simulink subsystem "PvtSubSys_VSM_LKA"  (R2020b)
settings: Solver=VariableStepAuto  StartTime=0.0  StopTime=10.0  RelTol=1e-3
values from neighbouring files (symbols this model uses):
  P_VSM_LKA_AbsEspInTime = 3.0    [LKA.sldd]
  P_VSM_LKA_absLongitudeAcceIn = 2.5    [LKA.sldd]
  P_VSM_LKA_absLongitudeAcceInTime = 3.0    [LKA.sldd]
  P_VSM_LKA_absLongitudeAcceOut = 3.0    [LKA.sldd]
  P_VSM_LKA_AccPedalPosnOut = 30.0    [LKA.sldd]
  P_VSM_LKA_AccPedalRateOutTime = 0.0    [LKA.sldd]
  P_VSM_LKA_AccRateIn = 30.0    [LKA.sldd]
  P_VSM_LKA_AccRateInTime = 1.5    [LKA.sldd]
  P_VSM_LKA_AccRateOut = 70.0    [LKA.sldd]
  P_VSM_LKA_BrakePressIn = 3.0    [LKA.sldd]
  P_VSM_LKA_BrakePressInTime = 1.5    [LKA.sldd]
  P_VSM_LKA_BrakePressOut = 5.0    [LKA.sldd]
  P_VSM_LKA_CurveFactor = 1.0    [LKA.sldd]
  P_VSM_LKA_DriverInputTrqValueIn = 2.0    [LKA.sldd]
  P_VSM_LKA_DriverInputTrqValueInTime = 3.0    [LKA.sldd]
  P_VSM_LKA_DriverInputTrqValueOut = 2.3    [LKA.sldd]
  P_VSM_LKA_EndSwitch = 1.0    [LKA.sldd]
  P_VSM_LKA_LaneChangeOffset = 0.11    [LKA.sldd]
  P_VSM_LKA_LaneCurveIn = 0.005    [LKA.sldd]
  P_VSM_LKA_LaneCurveOut = 0.006    [LKA.sldd]
  P_VSM_LKA_LateralAcceIn = 3.0    [LKA.sldd]
  P_VSM_LKA_LateralAcceInTime = 3.0    [LKA.sldd]
  P_VSM_LKA_LateralAcceOut = 3.5    [LKA.sldd]
  P_VSM_LKA_LongitudeAcceIn = 3.0    [LKA.sldd]
  P_VSM_LKA_LongitudeAcceOut = 3.5    [LKA.sldd]
  P_VSM_LKA_OverrideInTime = 1.5    [LKA.sldd]
  P_VSM_LKA_OverrideTime = 0.3    [LKA.sldd]
  P_VSM_LKA_OverrideValue = 1.2    [LKA.sldd]
  P_VSM_LKA_State_Absesp_enable = 1.0    [LKA.sldd]
  P_VSM_LKA_State_Accpedalrate_enable = 1.0    [LKA.sldd]
  P_VSM_LKA_State_Breakpressure_enable = 1.0    [LKA.sldd]
  P_VSM_LKA_State_DriverInputTrqValue_enable = 1.0    [LKA.sldd]
  P_VSM_LKA_State_Eps_enable = 1.0    [LKA.sldd]
  P_VSM_LKA_State_ESSSts_enable = 1.0    [LKA.sldd]
  P_VSM_LKA_State_Failsafe_enable = 1.0    [LKA.sldd]
  P_VSM_LKA_State_GEAR_enable = 1.0    [LKA.sldd]
  P_VSM_LKA_State_Handson_enable = 1.0    [LKA.sldd]
  P_VSM_LKA_State_Headingangle_enable = 1.0    [LKA.sldd]
  P_VSM_LKA_State_Lane_enable = 1.0    [LKA.sldd]
  P_VSM_LKA_State_LaneChange_enable = 1.0    [LKA.sldd]
  P_VSM_LKA_State_Lanecurve_enable = 1.0    [LKA.sldd]
  P_VSM_LKA_State_LateralAcce_enable = 1.0    [LKA.sldd]
  P_VSM_LKA_State_LongitudeAcc_enable = 1.0    [LKA.sldd]
  P_VSM_LKA_State_Overide_enable = 1.0    [LKA.sldd]
  P_VSM_LKA_State_Param_AngleOffset = 0.15    [LKA.sldd]
  P_VSM_LKA_State_Param_InterventionZoneIn = 0.4    [LKA.sldd]
  P_VSM_LKA_State_Param_InterventionZoneOut = -0.65    [LKA.sldd]
  P_VSM_LKA_State_Param_LaneCurve : value not decoded    [LKA.sldd]
  P_VSM_LKA_State_Param_LaneCurve_Offset : value not decoded    [LKA.sldd]
  P_VSM_LKA_State_Param_LaneWidth_Offset : value not decoded    [LKA.sldd]
  P_VSM_LKA_State_Param_OutOffset = 0.2    [LKA.sldd]
  P_VSM_LKA_State_Param_REInterventionZoneIn = 0.55    [LKA.sldd]
  P_VSM_LKA_State_Param_Sensitive_Offset : value not decoded    [LKA.sldd]
  P_VSM_LKA_State_SteerWheelAngle_enable = 1.0    [LKA.sldd]
  P_VSM_LKA_State_SteerWheelSpd_enable = 1.0    [LKA.sldd]
  P_VSM_LKA_State_TJASts_enable = 1.0    [LKA.sldd]
  P_VSM_LKA_State_TurnLight_enable = 1.0    [LKA.sldd]
  P_VSM_LKA_State_Vehspeed_enable = 1.0    [LKA.sldd]
  P_VSM_LKA_State_Yawsup_enable = 1.0    [LKA.sldd]
  P_VSM_LKA_SteerWheelAngleIn = 70.0    [LKA.sldd]
  P_VSM_LKA_SteerWheelAngleInTime = 3.0    [LKA.sldd]
  P_VSM_LKA_SteerWheelAngleOut = 90.0    [LKA.sldd]
  P_VSM_LKA_SteerWheelSpdIn = 150.0    [LKA.sldd]
  P_VSM_LKA_SteerWheelSpdInTime = 3.0    [LKA.sldd]
  P_VSM_LKA_SteerWheelSpdOut = 200.0    [LKA.sldd]
  P_VSM_LKA_TurnLightInTime = 3.0    [LKA.sldd]
  P_VSM_LKA_Warnarea1 = -0.55    [LKA.sldd]
  P_VSM_LKA_Warnarea2 = -0.35    [LKA.sldd]
  P_VSM_LKA_WarnInTime = 2.0    [LKA.sldd]
  P_VSM_LKA_WhelDy = 2.0    [LKA.sldd]
  P_VSM_LKA_YawRateIn = 0.2    [LKA.sldd]
  P_VSM_LKA_YawRateInTime = 1.0    [LKA.sldd]
  P_VSM_LKA_YawRateOut = 0.25    [LKA.sldd]
undefined symbols (not defined in the file or in its folder): P_VSM_LKA_AddOffset, P_VSM_LSMC_SampleTime, STATE
libraries: simulink x162
(part 1 of 5)
settings Model: Creator=GW00133806  LastModifiedBy=GW00199575

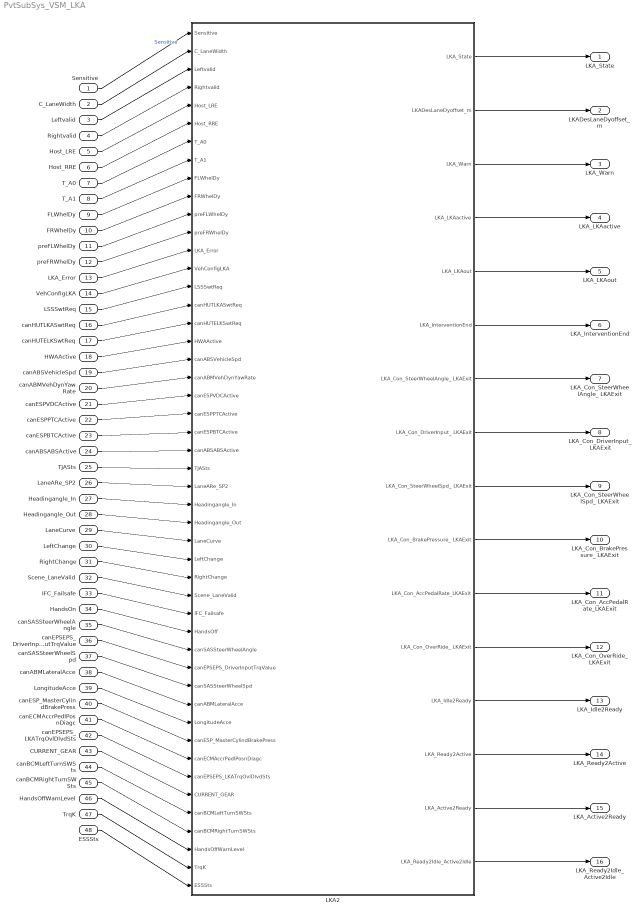
== system PvtSubSys_VSM_LKA ==
  Sensitive : Inport  OutDataTypeStr=uint8
  C_LaneWidth : Inport  Port=2  OutDataTypeStr=single
  Leftvalid : Inport  Port=3  OutDataTypeStr=boolean
  Rightvalid : Inport  Port=4  OutDataTypeStr=boolean
  Host_LRE : Inport  Port=5  OutDataTypeStr=boolean
  Host_RRE : Inport  Port=6  OutDataTypeStr=boolean
  T_A0 : Inport  Port=7  OutDataTypeStr=single
  T_A1 : Inport  Port=8  OutDataTypeStr=single
  FLWhelDy : Inport  Port=9  OutDataTypeStr=single
  FRWhelDy : Inport  Port=10  OutDataTypeStr=single
  preFLWhelDy : Inport  Port=11  OutDataTypeStr=single
  preFRWhelDy : Inport  Port=12  OutDataTypeStr=single
  LKA_Error : Inport  Port=13  OutDataTypeStr=uint8
  VehConfigLKA : Inport  Port=14  OutDataTypeStr=uint8
  LSSSwtReq : Inport  Port=15  OutDataTypeStr=boolean
  canHUTLKASwtReq : Inport  Port=16  OutDataTypeStr=boolean
  canHUTELKSwtReq : Inport  Port=17  OutDataTypeStr=boolean
  HWAActive : Inport  Port=18  OutDataTypeStr=boolean
  canABSVehicleSpd : Inport  Port=19  OutDataTypeStr=single
  canABMVehDynYawRate : Inport  Port=20  OutDataTypeStr=single
  canESPVDCActive : Inport  Port=21  OutDataTypeStr=boolean
  canESPPTCActive : Inport  Port=22  OutDataTypeStr=boolean
  canESPBTCActive : Inport  Port=23  OutDataTypeStr=boolean
  canABSABSActive : Inport  Port=24  OutDataTypeStr=boolean
  TJASts : Inport  Port=25  OutDataTypeStr=uint8
  LaneARe_SP2 : Inport  Port=26  OutDataTypeStr=Bus: LaneARe_SP_LKA
  Headingangle_In : Inport  Port=27  OutDataTypeStr=boolean
  Headingangle_Out : Inport  Port=28  OutDataTypeStr=boolean
  LaneCurve : Inport  Port=29  OutDataTypeStr=single
  LeftChange : Inport  Port=30  OutDataTypeStr=boolean
  RightChange : Inport  Port=31  OutDataTypeStr=boolean
  Scene_LaneValid : Inport  Port=32  OutDataTypeStr=single
  IFC_Failsafe : Inport  Port=33  OutDataTypeStr=double
  HandsOn : Inport  Port=34  OutDataTypeStr=boolean
  canSASSteerWheelAngle : Inport  Port=35  OutDataTypeStr=single
  canEPSEPS_DriverInputTrqValue : Inport  Port=36  OutDataTypeStr=single
  canSASSteerWheelSpd : Inport  Port=37  OutDataTypeStr=single
  canABMLateralAcce : Inport  Port=38  OutDataTypeStr=single
  LongitudeAcce : Inport  Port=39  OutDataTypeStr=single
  canESP_MasterCylindBrakePress : Inport  Port=40  OutDataTypeStr=single
  canECMAccrPedlPosnDiagc : Inport  Port=41  OutDataTypeStr=single
  canEPSEPS_LKATrqOvlDlvdSts : Inport  Port=42  OutDataTypeStr=uint8
  CURRENT_GEAR : Inport  Port=43  OutDataTypeStr=uint8
  canBCMLeftTurnSWSts : Inport  Port=44  OutDataTypeStr=boolean
  canBCMRightTurnSWSts : Inport  Port=45  OutDataTypeStr=boolean
  HandsOffWarnLevel : Inport  Port=46  OutDataTypeStr=uint8
  TrqK : Inport  Port=47  OutDataTypeStr=single
  ESSSts : Inport  Port=48  OutDataTypeStr=uint8
  LKA2 : Subsystem
  LKA_State : Outport
  LKADesLaneDyoffset_m : Outport  Port=2
  LKA_Warn : Outport  Port=3
  LKA_LKAactive : Outport  Port=4
  LKA_LKAout : Outport  Port=5
  LKA_InterventionEnd : Outport  Port=6
  LKA_Con_SteerWheelAngle_ LKAExit : Outport  Port=7
  LKA_Con_DriverInput_ LKAExit : Outport  Port=8
  LKA_Con_SteerWheelSpd_ LKAExit : Outport  Port=9
  LKA_Con_BrakePressure_ LKAExit : Outport  Port=10
  LKA_Con_AccPedalRate_LKAExit : Outport  Port=11
  LKA_Con_OverRide_ LKAExit : Outport  Port=12
  LKA_Idle2Ready : Outport  Port=13
  LKA_Ready2Active : Outport  Port=14
  LKA_Active2Ready : Outport  Port=15
  LKA_Ready2Idle_Active2Idle : Outport  Port=16
  wires:
  IFC_Failsafe/1 -> LKA2/33(IFC_Failsafe)
  Scene_LaneValid/1 -> LKA2/32(Scene_LaneValid)
  LeftChange/1 -> LKA2/30(LeftChange)
  canECMAccrPedlPosnDiagc/1 -> LKA2/41(canECMAccrPedlPosnDiagc)
  RightChange/1 -> LKA2/31(RightChange)
  canABSVehicleSpd/1 -> LKA2/19(canABSVehicleSpd)
  HandsOffWarnLevel/1 -> LKA2/46(HandsOffWarnLevel)
  canBCMRightTurnSWSts/1 -> LKA2/45(canBCMRightTurnSWSts)
  CURRENT_GEAR/1 -> LKA2/43(CURRENT_GEAR)
  LaneCurve/1 -> LKA2/29(LaneCurve)
  FLWhelDy/1 -> LKA2/9(FLWhelDy)
  LKA2/8(LKA_Con_DriverInput_ LKAExit) -> LKA_Con_DriverInput_ LKAExit/1
  ESSSts/1 -> LKA2/48(ESSSts)
  canBCMLeftTurnSWSts/1 -> LKA2/44(canBCMLeftTurnSWSts)
  HandsOn/1 -> LKA2/34(HandsOff)
  LaneARe_SP2/1 -> LKA2/26(LaneARe_SP2)
  canESP_MasterCylindBrakePress/1 -> LKA2/40(canESP_MasterCylindBrakePress)
  LKA2/5(LKA_LKAout) -> LKA_LKAout/1
  LongitudeAcce/1 -> LKA2/39(LongitudeAcce)
  LKA2/16(LKA_Ready2Idle_Active2Idle) -> LKA_Ready2Idle_Active2Idle/1
  LKA2/15(LKA_Active2Ready) -> LKA_Active2Ready/1
  canABMLateralAcce/1 -> LKA2/38(canABMLateralAcce)
  canEPSEPS_DriverInputTrqValue/1 -> LKA2/36(canEPSEPS_DriverInputTrqValue)
  Headingangle_Out/1 -> LKA2/28(Headingangle_Out)
  LKA2/9(LKA_Con_SteerWheelSpd_ LKAExit) -> LKA_Con_SteerWheelSpd_ LKAExit/1
  canEPSEPS_LKATrqOvlDlvdSts/1 -> LKA2/42(canEPSEPS_LKATrqOvlDlvdSts)
  LKA2/2(LKADesLaneDyoffset_m) -> LKADesLaneDyoffset_m/1
  HWAActive/1 -> LKA2/18(HWAActive)
  canSASSteerWheelSpd/1 -> LKA2/37(canSASSteerWheelSpd)
  Headingangle_In/1 -> LKA2/27(Headingangle_In)
  canESPPTCActive/1 -> LKA2/22(canESPPTCActive)
  canABSABSActive/1 -> LKA2/24(canABSABSActive)
  preFLWhelDy/1 -> LKA2/11(preFLWhelDy)
  LSSSwtReq/1 -> LKA2/15(LSSSwtReq)
  canESPBTCActive/1 -> LKA2/23(canESPBTCActive)
  LKA2/13(LKA_Idle2Ready) -> LKA_Idle2Ready/1
  canESPVDCActive/1 -> LKA2/21(canESPVDCActive)
  LKA2/1(LKA_State) -> LKA_State/1
  Host_LRE/1 -> LKA2/5(Host_LRE)
  LKA2/11(LKA_Con_AccPedalRate_LKAExit) -> LKA_Con_AccPedalRate_LKAExit/1
  preFRWhelDy/1 -> LKA2/12(preFRWhelDy)
  LKA2/6(LKA_InterventionEnd) -> LKA_InterventionEnd/1
  canHUTLKASwtReq/1 -> LKA2/16(canHUTLKASwtReq)
  VehConfigLKA/1 -> LKA2/14(VehConfigLKA)
  LKA_Error/1 -> LKA2/13(LKA_Error)
  canABMVehDynYawRate/1 -> LKA2/20(canABMVehDynYawRate)
  LKA2/4(LKA_LKAactive) -> LKA_LKAactive/1
  Rightvalid/1 -> LKA2/4(Rightvalid)
  LKA2/7(LKA_Con_SteerWheelAngle_ LKAExit) -> LKA_Con_SteerWheelAngle_ LKAExit/1
  Host_RRE/1 -> LKA2/6(Host_RRE)
  LKA2/10(LKA_Con_BrakePressure_ LKAExit) -> LKA_Con_BrakePressure_ LKAExit/1
  Leftvalid/1 -> LKA2/3(Leftvalid)
  C_LaneWidth/1 -> LKA2/2(C_LaneWidth)
  T_A1/1 -> LKA2/8(T_A1)
  FRWhelDy/1 -> LKA2/10(FRWhelDy)
  Sensitive/1 -> LKA2/1(Sensitive)  "Sensitive"
  canSASSteerWheelAngle/1 -> LKA2/35(canSASSteerWheelAngle)
  TrqK/1 -> LKA2/47(TrqK)
  T_A0/1 -> LKA2/7(T_A0)
  LKA2/12(LKA_Con_OverRide_ LKAExit) -> LKA_Con_OverRide_ LKAExit/1
  LKA2/3(LKA_Warn) -> LKA_Warn/1
  LKA2/14(LKA_Ready2Active) -> LKA_Ready2Active/1
  canHUTELKSwtReq/1 -> LKA2/17(canHUTELKSwtReq)
  TJASts/1 -> LKA2/25(TJASts)

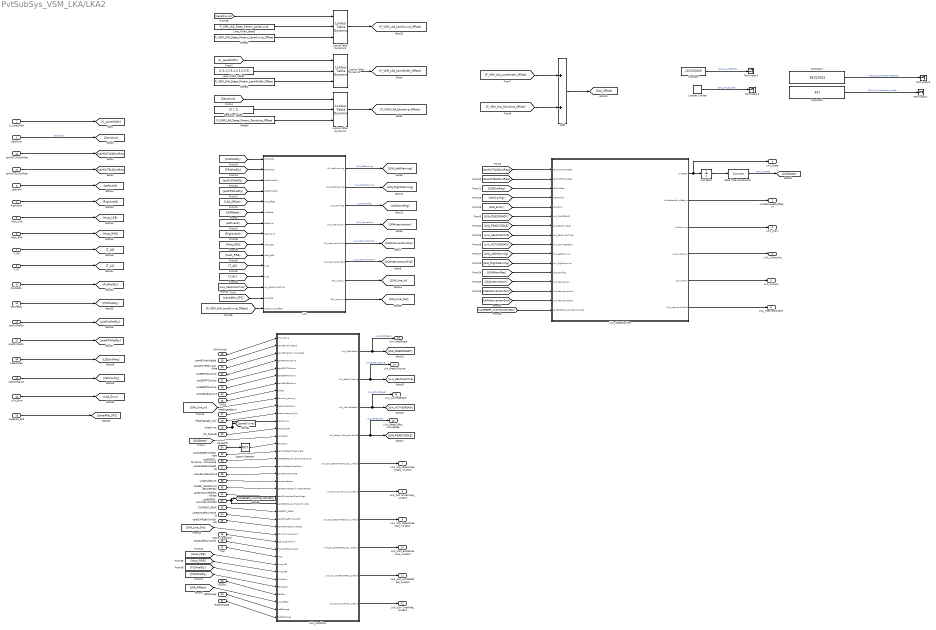
== system PvtSubSys_VSM_LKA/LKA2 ==
  Sensitive : Inport  OutDataTypeStr=uint8
  C_LaneWidth : Inport  Port=2  OutDataTypeStr=single
  Leftvalid : Inport  Port=3  OutDataTypeStr=boolean
  Rightvalid : Inport  Port=4  OutDataTypeStr=boolean
  Host_LRE : Inport  Port=5  OutDataTypeStr=boolean
  Host_RRE : Inport  Port=6  OutDataTypeStr=boolean
  T_A0 : Inport  Port=7  OutDataTypeStr=single
  T_A1 : Inport  Port=8  OutDataTypeStr=single
  FLWhelDy : Inport  Port=9  OutDataTypeStr=single
  FRWhelDy : Inport  Port=10  OutDataTypeStr=single
  preFLWhelDy : Inport  Port=11  OutDataTypeStr=single
  preFRWhelDy : Inport  Port=12  OutDataTypeStr=single
  LKA_Error : Inport  Port=13  OutDataTypeStr=uint8
  VehConfigLKA : Inport  Port=14  OutDataTypeStr=uint8
  LSSSwtReq : Inport  Port=15  OutDataTypeStr=boolean
  canHUTLKASwtReq : Inport  Port=16  OutDataTypeStr=boolean
  canHUTELKSwtReq : Inport  Port=17  OutDataTypeStr=boolean
  HWAActive : Inport  Port=18  OutDataTypeStr=boolean
  canABSVehicleSpd : Inport  Port=19  OutDataTypeStr=single
  canABMVehDynYawRate : Inport  Port=20  OutDataTypeStr=single
  canESPVDCActive : Inport  Port=21  OutDataTypeStr=boolean
  canESPPTCActive : Inport  Port=22  OutDataTypeStr=boolean
  canESPBTCActive : Inport  Port=23  OutDataTypeStr=boolean
  canABSABSActive : Inport  Port=24  OutDataTypeStr=boolean
  TJASts : Inport  Port=25
  LaneARe_SP2 : Inport  Port=26
  Headingangle_In : Inport  Port=27  OutDataTypeStr=boolean
  Headingangle_Out : Inport  Port=28  OutDataTypeStr=boolean
  LaneCurve : Inport  Port=29  OutDataTypeStr=single
  LeftChange : Inport  Port=30  OutDataTypeStr=boolean
  RightChange : Inport  Port=31  OutDataTypeStr=boolean
  Scene_LaneValid : Inport  Port=32  OutDataTypeStr=single
  IFC_Failsafe : Inport  Port=33  OutDataTypeStr=double
  HandsOff : Inport  Port=34  OutDataTypeStr=boolean
  canSASSteerWheelAngle : Inport  Port=35  OutDataTypeStr=single
  canEPSEPS_DriverInputTrqValue : Inport  Port=36  OutDataTypeStr=single
  canSASSteerWheelSpd : Inport  Port=37  OutDataTypeStr=single
  canABMLateralAcce : Inport  Port=38  OutDataTypeStr=single
  LongitudeAcce : Inport  Port=39  OutDataTypeStr=single
  canESP_MasterCylindBrakePress : Inport  Port=40  OutDataTypeStr=single
  canECMAccrPedlPosnDiagc : Inport  Port=41  OutDataTypeStr=single
  canEPSEPS_LKATrqOvlDlvdSts : Inport  Port=42  OutDataTypeStr=uint8
  CURRENT_GEAR : Inport  Port=43  OutDataTypeStr=uint8
  canBCMLeftTurnSWSts : Inport  Port=44  OutDataTypeStr=boolean
  canBCMRightTurnSWSts : Inport  Port=45  OutDataTypeStr=boolean
  HandsOffWarnLevel : Inport  Port=46  OutDataTypeStr=uint8
  TrqK : Inport  Port=47  OutDataTypeStr=single
  ESSSts : Inport  Port=48  OutDataTypeStr=uint8
  Add1 : Sum
  Constant : Constant  Value=2103150406  OutDataTypeStr=uint32
  Constant1 : Constant  Value=38252004  OutDataTypeStr=uint32
  Constant2 : Constant  Value=301  OutDataTypeStr=uint16
  Counter Limited : simulink/Sources/Counter Limited  uplimit=7  tsamp=-1
  Data Type Conversion2 : DataTypeConversion
  LKA : Subsystem
  LKA_Condition : Subsystem
  LKA_StateMachine : Subsystem
  Lane_Width_table1 : Constant  Value=[2.5,3,3.5,4,4.5,5,5.5]
  Lane_Width_table2 : Constant  Value=P_VSM_LKA_State_Param_LaneCurve
  Logical Operator : Logic  Operator=NOT  AllPortsSameDT=off  OutDataTypeStr=boolean
  Lookup Table Dynamic1 : simulink/Lookup Tables/Lookup Table Dynamic  LookUpMeth=Interpolation-Use End Values  OutDataType=fixdt('double')  OutScaling=[]  OutputDataTypeScalingMode=Specify via dialog  OutDataTypeStr=double  DoSatur=off
  Lookup Table Dynamic2 : simulink/Lookup Tables/Lookup Table Dynamic  LookUpMeth=Interpolation-Use End Values  OutDataType=fixdt('double')  OutScaling=[]  OutputDataTypeScalingMode=Specify via dialog  OutDataTypeStr=double  DoSatur=off
  Lookup Table Dynamic3 : simulink/Lookup Tables/Lookup Table Dynamic  LookUpMeth=Interpolation-Use End Values  OutDataType=fixdt('double')  OutScaling=[]  OutputDataTypeScalingMode=Specify via dialog  OutDataTypeStr=double  DoSatur=off
  Offset1 : Constant  Value=P_VSM_LKA_State_Param_LaneWidth_Offset
  Offset2 : Constant  Value=P_VSM_LKA_State_Param_LaneCurve_Offset
  Offset4 : Constant  Value=P_VSM_LKA_State_Param_Sensitive_Offset
  Sensitive_table2 : Constant  Value=[0 1 2]
  Terminator{3..4,6..7} (4 alike) : Terminator
  Unit Delay : UnitDelay  InitialCondition=STATE.OFF  SampleTime=-1  HasFrameUpgradeWarning=on
  LKA_State : Outport
  LKADesLaneDyoffset_m : Outport  Port=2
  LKA_Warn : Outport  Port=3
  LKA_LKAactive : Outport  Port=4
  LKA_LKAout : Outport  Port=5
  LKA_InterventionEnd : Outport  Port=6
  LKA_Con_SteerWheelAngle_ LKAExit : Outport  Port=7
  LKA_Con_DriverInput_ LKAExit : Outport  Port=8
  LKA_Con_SteerWheelSpd_ LKAExit : Outport  Port=9
  LKA_Con_BrakePressure_ LKAExit : Outport  Port=10
  LKA_Con_AccPedalRate_LKAExit : Outport  Port=11
  LKA_Con_OverRide_ LKAExit : Outport  Port=12
  LKA_Idle2Ready : Outport  Port=13
  LKA_Ready2Active : Outport  Port=14
  LKA_Active2Ready : Outport  Port=15
  LKA_Ready2Idle_Active2Idle : Outport  Port=16
  wires:
  [canEPSEPS_LKATrqOvlDlvdSts] -> LKA_StateMachine/16(canEPSEPS_LKATrqOvlDlvdSts)
  canEPSEPS_LKATrqOvlDlvdSts/1 -> [canEPSEPS_LKATrqOvlDlvdSts], LKA_Condition/23(canEPSEPS_LKATrqOvlDlvdSts)
  LKA/8(ELK_Lane_out) -> [LKA_Line_Out]
  LKA/7(ELK_Lane_in) -> [LKA_Line_In]
  [LaneARe_SP2] -> LKA/14(LaneARe)
  LaneARe_SP2/1 -> [LaneARe_SP2]
  Constant/1 -> Terminator3/1  "VSM_LKA_VERSION"
  Counter Limited/1 -> Terminator4/1  "VSM_LKA_Counter"
  TJASts/1 -> LKA_Condition/8(TJASts)
  Logical Operator/1 -> LKA_Condition/15(HandsOn)
  LKA_Condition/5(LKA_Con_SteerWheelAngle_ LKAExit) -> LKA_Con_SteerWheelAngle_ LKAExit/1
  canABSABSActive/1 -> LKA_Condition/7(canABSABSActive)
  LKA_StateMachine/6(LKA_InterventionEnd) -> LKA_InterventionEnd/1
  LKA_StateMachine/5(LKA_LKAout) -> LKA_LKAout/1
  LKA_Condition/3(LKA_Active2Ready) -> LKA_Active2Ready/1, [LKA_ACTIVE2READY]  "LKA_Active2Ready"
  [LKAInterventionEnd] -> LKA_StateMachine/15(LKAInterventionEnd)
  LKA/1(LKA_LeftWarning) -> [LKA_LeftWarning]  "LKA_LeftWarning"
  LKA_Condition/8(LKA_Con_BrakePressure_ LKAExit) -> LKA_Con_BrakePressure_ LKAExit/1
  LKA/3(LKA_Warnflag) -> [LKAWarnflag]  "LKA_Warnflag"
  TrqK/1 -> LKA_Condition/30(TrqK)
  canABMLateralAcce/1 -> LKA_Condition/19(canABMLateralAcce)
  HandsOffWarnLevel/1 -> LKA_Condition/29(HandsOffWarnLevel)
  canABSVehicleSpd/1 -> LKA_Condition/2(canABSVehicleSpd)
  canSASSteerWheelAngle/1 -> LKA_Condition/16(canSASSteerWheelAngle)
  [Rightvalid] -> LKA/8(RightValid)
  preFRWhelDy/1 -> [preFRWhelDy]
  [LKA_READY2IDLE] -> LKA_StateMachine/7(LKA_READY2IDLE)
  LKA_Condition/9(LKA_Con_AccPedalRate_LKAExit) -> LKA_Con_AccPedalRate_LKAExit/1
  Host_RRE/1 -> [Host_RRE]
  canESP_MasterCylindBrakePress/1 -> LKA_Condition/21(canESP_MasterCylindBrakePress)
  LKA_Condition/6(LKA_Con_DriverInput_ LKAExit) -> LKA_Con_DriverInput_ LKAExit/1
  Unit Delay/1 -> Data Type Conversion2/1
  Data Type Conversion2/1 -> [LKAState]  "VSM_LKAState"
  Headingangle_In/1 -> LKA_Condition/10(Headingangle_In)
  canHUTLKASwtReq/1 -> [canHUTLKASwtReq]
  T_A1/1 -> [T_A1]
  Lookup Table Dynamic1/1 -> [P_VSM_LKA_LaneWidth_Offset]
  Headingangle_Out/1 -> LKA_Condition/11(Headingangle_Out)
  [LKA_READY2ACTIVE] -> LKA_StateMachine/8(LKA_READY2ACTIVE)
  [Host_RRE] -> LKA_Condition/32(Host_RRE)
  [FRWhelDy] -> LKA_Condition/34(FRWhelDy)
  Host_LRE/1 -> [Host_LRE]
  LKA_StateMachine/2(LKADesLaneDyoffset_m) -> LKADesLaneDyoffset_m/1
  [LKA_Offset] -> LKA/5(LKA_Offset)
  Lookup Table Dynamic2/1 -> [P_VSM_LKA_Sensitive_Offset]
  Leftvalid/1 -> [Leftvalid]
  HWAActive/1 -> LKA_Condition/1(HWAActive)
  LKA_Condition/4(LKA_Ready2Idle_Active2Idle) -> LKA_Ready2Idle_Active2Idle/1, [LKA_READY2IDLE]  "LKA_Other2Idle"
  canBCMLeftTurnSWSts/1 -> LKA_Condition/25(canBCMLeftTurnSWSts)
  FLWhelDy/1 -> [FLWhelDy]
  [Leftvalid] -> LKA/7(LeftValid)
  LeftChange/1 -> LKA_Condition/37(LeftChange)
  RightChange/1 -> LKA_Condition/38(RightChange)
  [LKA_RightWarning] -> LKA_StateMachine/11(LKA_RightWarning)
  preFLWhelDy/1 -> [preFLWhelDy]
  [FLWhelDy] -> LKA_Condition/33(FLWhelDy)
  LKA_Error/1 -> [LKA_Error]
  [LKA_Offset] -> LKA_Condition/36(LKA_Offset)
  LKA_Condition/10(LKA_Con_OverRide_ LKAExit) -> LKA_Con_OverRide_ LKAExit/1
  canESPBTCActive/1 -> LKA_Condition/6(canESPBTCActive)
  LKA/6(LKA_InterventionEnd) -> [LKAInterventionEnd]  "LKA_InterventionEnd"
  Rightvalid/1 -> [Rightvalid]
  [LKA_IDLE2READY] -> LKA_StateMachine/6(LKA_IDLE2READY)
  [C_LaneWidth] -> Lookup Table Dynamic1/1
  canBCMRightTurnSWSts/1 -> LKA_Condition/26(canBCMRightTurnSWSts)
  Sensitive_table2/1 -> Lookup Table Dynamic2/2
  LaneCurve/1 -> [LaneCurve], LKA_Condition/12(LaneCurve)
  VehConfigLKA/1 -> [VehConfig]
  Scene_LaneValid/1 -> LKA_Condition/28(Scene_LaneValid)
  [T_A1] -> LKA/12(T_A1)
  [canHUTLKASwtReq] -> LKA_StateMachine/1(canHUTLKASwtReq)
  canHUTELKSwtReq/1 -> [canHUTELKSwtReq]
  Add1/1 -> [LKA_Offset]
  LKA_Condition/7(LKA_Con_SteerWheelSpd_ LKAExit) -> LKA_Con_SteerWheelSpd_ LKAExit/1
  [preFRWhelDy] -> LKA/4(preFRWhelDy)
  [LKA_ACTIVE2READY] -> LKA_StateMachine/9(LKA_ACTIVE2READY)
  [preFLWhelDy] -> LKA/3(preFLWhelDy)
  [Sensitive] -> Lookup Table Dynamic2/1
  canESPVDCActive/1 -> LKA_Condition/4(canESPVDCActive)
  Offset4/1 -> Lookup Table Dynamic2/3
  [canHUTELKSwtReq] -> LKA_StateMachine/2(canHUTELKSwtReq)
  LKA/2(LKA_RightWarning) -> [LKA_RightWarning]  "LKA_RightWarning"
  [Host_RRE] -> LKA/10(Host_RRE)
  canECMAccrPedlPosnDiagc/1 -> LKA_Condition/22(canECMAccrPedlPosnDiagc)
  LKA_Condition/2(LKA_Ready2Active) -> LKA_Ready2Active/1, [LKA_READY2ACTIVE]  "LKA_Ready2Active"
  canABMVehDynYawRate/1 -> LKA_Condition/3(canABMVehDynYawRate2)
  CURRENT_GEAR/1 -> LKA_Condition/24(CURRENT_GEAR)
  Sensitive/1 -> [Sensitive]  "Sensitive"
  [LKAWarnflag] -> LKA_StateMachine/12(LKAWarnflag)
  HandsOff/1 -> Logical Operator/1
  canSASSteerWheelSpd/1 -> LKA_Condition/18(canSASSteerWheelSpd)
  canEPSEPS_DriverInputTrqValue/1 -> LKA_Condition/17(canEPSEPS_DriverInputTrqValue)
  [P_VSM_LKA_Sensitive_Offset] -> Add1/2
  LKA_StateMachine/4(LKA_LKAactive) -> LKA_LKAactive/1
  [VehConfig] -> LKA_StateMachine/4(VehConfig)
  LKA/4(LKA_Intervention) -> [LKAIntervention]  "LKA_Intervention"
  [LKA_LeftWarning] -> LKA_StateMachine/10(LKA_LeftWarning)
  [T_A0] -> LKA/11(T_A0)
  [P_VSM_LKA_LaneWidth_Offset] -> Add1/1
  ESSSts/1 -> LKA_Condition/35(ESSSts)
  [LKA_Error] -> LKA_StateMachine/5(LKA_Error)
  LongitudeAcce/1 -> LKA_Condition/20(LongitudeAcce)
  C_LaneWidth/1 -> [C_LaneWidth]
  [LKA_READY2ACTIVE] -> LKA/13(LKA_READY2ACTIVE)
  [LKA_Line_In] -> LKA_Condition/9(Common_Lane_in)
  LKA_StateMachine/1(LKAState) -> LKA_State/1, Unit Delay/1
  [LKAState] -> LKA/6(LKAState)
  [LKAState] -> LKA_Condition/14(LKA_State)
  LKA_Condition/1(LKA_Idle2Ready) -> LKA_Idle2Ready/1, [LKA_IDLE2READY]  "LKA_Idle2Ready"
  [Host_LRE] -> LKA_Condition/31(Host_LRE)
  Lane_Width_table1/1 -> Lookup Table Dynamic1/2
  LSSSwtReq/1 -> [LSSSwtReq]
  LKA_StateMachine/3(LKAWarning) -> LKA_Warn/1
  [LKAIntervention] -> LKA_StateMachine/13(LKAIntervention)
  FRWhelDy/1 -> [FRWhelDy]
  canESPPTCActive/1 -> LKA_Condition/5(canESPPTCActive)
  LKA/5(LKA_InterventionOut) -> [LKAInterventionOut]  "LKA_InterventionOut"
  [LKAInterventionOut] -> LKA_StateMachine/14(LKAInterventionOut)
  [LSSSwtReq] -> LKA_StateMachine/3(LSSSwtReq)
  [FRWhelDy] -> LKA/2(FRWhelDy)
  [Host_LRE] -> LKA/9(Host_LRE)
  [LKA_Line_Out] -> LKA_Condition/27(Common_Lane_Out)
  T_A0/1 -> [T_A0]
  IFC_Failsafe/1 -> LKA_Condition/13(IFC_Failsafe)
  Offset1/1 -> Lookup Table Dynamic1/3
  [FLWhelDy] -> LKA/1(FLWhelDy)
  [LaneCurve] -> Lookup Table Dynamic3/1
  Offset2/1 -> Lookup Table Dynamic3/3
  Lane_Width_table2/1 -> Lookup Table Dynamic3/2
  Lookup Table Dynamic3/1 -> [P_VSM_LKA_LaneCurve_Offset]
  Constant1/1 -> Terminator6/1  "VSM_LKA_SubModel_VERSION"
  Constant2/1 -> Terminator7/1  "VSM_LKA_SubModel_Number"
  [P_VSM_LKA_LaneCurve_Offset] -> LKA/15(LaneCurve_Offset)
